simulink model "ex3"  (R2023b)
settings: Solver=ode3  StartTime=0.0  StopTime=40.0  FixedStep=0.0001  RelTol=1e-3
libraries: simulink_extras x8
settings Model: Creator=Andrei  LastModifiedBy=Andrei

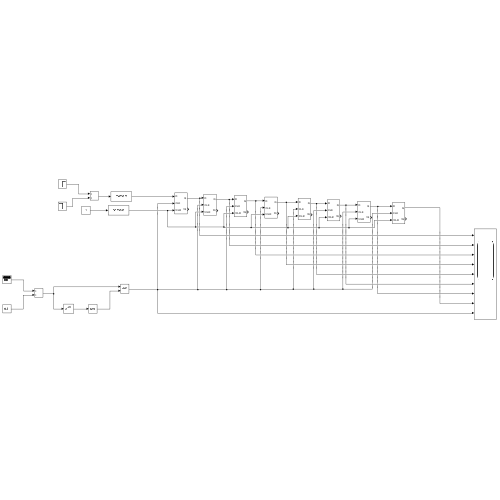
[thumbnail: Simulink's stored preview of the top-level diagram]
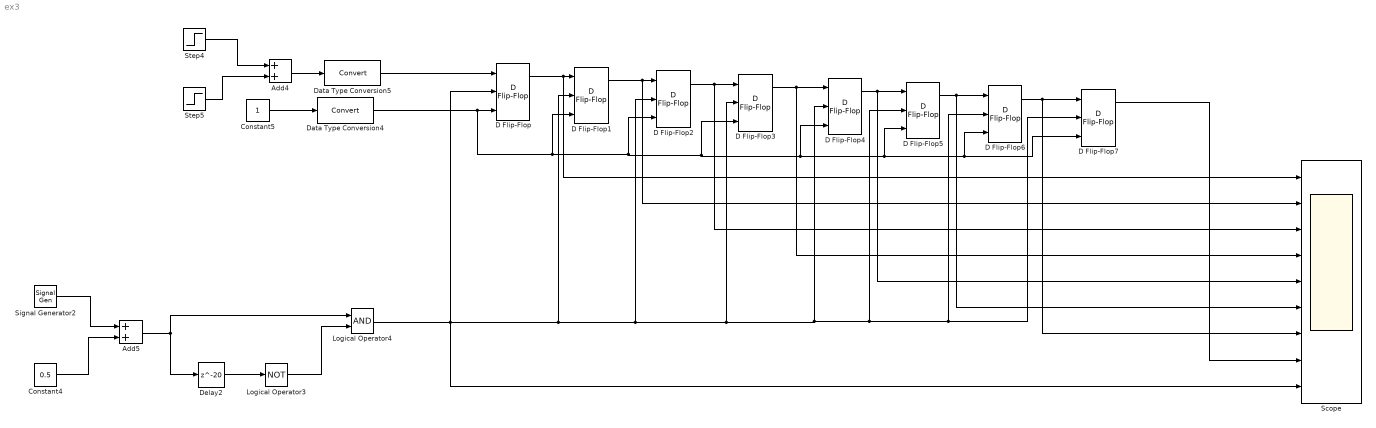
== system ex3 ==
  Add4 : Sum
  Add5 : Sum
  Constant4 : Constant  Value=0.5
  Constant5 : Constant
  D Flip-Flop{,1..7} (8 alike) : simulink_extras/Flip Flops/D Flip-Flop
  Data Type Conversion4 : DataTypeConversion  SaturateOnIntegerOverflow=off  RndMeth=Floor
  Data Type Conversion5 : DataTypeConversion  SaturateOnIntegerOverflow=off  RndMeth=Floor
  Delay2 : Delay  DelayLength=20  InitialCondition=0
  Logical Operator3 : Logic  Operator=NOT  AllPortsSameDT=off  OutDataTypeStr=boolean
  Logical Operator4 : Logic  AllPortsSameDT=off  OutDataTypeStr=boolean
  Scope : Scope  NumInputPorts=9
  Signal Generator2 : SignalGenerator  WaveForm=square  Amplitude=0.5  Frequency=0.5
  Step4 : Step  Time=2.5
  Step5 : Step  Time=5.5  After=-1
  wires:
  Logical Operator4/1 -> D Flip-Flop7/2, D Flip-Flop6/2, D Flip-Flop5/2, D Flip-Flop4/2, D Flip-Flop3/2, D Flip-Flop2/2, D Flip-Flop1/2, D Flip-Flop/2, Scope/9
  D Flip-Flop/1 -> Scope/1, D Flip-Flop1/1
  D Flip-Flop1/1 -> Scope/2, D Flip-Flop2/1
  D Flip-Flop3/1 -> Scope/4, D Flip-Flop4/1
  D Flip-Flop4/1 -> Scope/5, D Flip-Flop5/1
  D Flip-Flop5/1 -> Scope/6, D Flip-Flop6/1
  D Flip-Flop6/1 -> Scope/7, D Flip-Flop7/1
  D Flip-Flop2/1 -> Scope/3, D Flip-Flop3/1
  D Flip-Flop7/1 -> Scope/8
  Data Type Conversion5/1 -> D Flip-Flop/1
  Data Type Conversion4/1 -> D Flip-Flop2/3, D Flip-Flop3/3, D Flip-Flop4/3, D Flip-Flop5/3, D Flip-Flop7/3, D Flip-Flop6/3, D Flip-Flop1/3, D Flip-Flop/3
  Add4/1 -> Data Type Conversion5/1
  Step4/1 -> Add4/1
  Constant5/1 -> Data Type Conversion4/1
  Signal Generator2/1 -> Add5/1
  Delay2/1 -> Logical Operator3/1
  Add5/1 -> Logical Operator4/1, Delay2/1
  Step5/1 -> Add4/2
  Constant4/1 -> Add5/2
  Logical Operator3/1 -> Logical Operator4/2
